simulink model "genpath_firmware"  (R2021a)
settings: Solver=FixedStepDiscrete  StartTime=0.0  StopTime=Inf  FixedStep=50e-6  RelTol=1e-3  EnableMultiTasking=on
undefined symbols (not defined in the file or in its folder): Down, GPTRIP1SEL, HW_BLDC_LQ, HW_BLDC_RS, TZ1, Up
libraries: c2802xlib x10, mcbcontrolslib x4, simulink x2, c280xlib x2, c28004xlib x2, dspstat3 x2, c2000lib x1
settings Model: SimulationMode=external  ExtModeTrigDuration=8  Creator=61301765  LastModifiedBy=61301765
settings OptimizationCC: DefaultUnderspecifiedDataType=single  EnhancedBackFolding=on  PassReuseOutputArgsAs=Individual arguments  ZeroExternalMemoryAtStartup=off  ZeroInternalMemoryAtStartup=off  MaxStackSize=1024  OptimizeBlockOrder=speed  DifferentSizesBufferReuse=on  OptimizationCustomize=off  DenormalBehavior=FlushToZero  EfficientTunableParamExpr=on
settings DebuggingCC: SignalRangeChecking=warning  ParameterPrecisionLossMsg=none  ParameterTunabilityLossMsg=error
settings HardwareCC: ProdBitPerChar=16  ProdBitPerInt=16  ProdBitPerPointer=32  ProdBitPerSizeT=32  ProdBitPerPtrDiffT=32  ProdLargestAtomicInteger=Integer  ProdLargestAtomicFloat=None  ProdWordSize=16  ProdLongLongMode=on  ProdHWDeviceType=Texas Instruments->C2000
settings SFSimCC: MATLABDynamicMemAlloc=off
settings RTWCC: SystemTargetFile=ert.tlc  HardwareBoard=TI Piccolo F280049C LaunchPad  TemplateMakefile=ert_default_tmf  Toolchain=Texas Instruments Code Composer Studio (C2000)
settings CodeAppCC: ForceParamTrailComments=on  IgnoreCustomStorageClasses=off  OperatorAnnotations=on  SimulinkDataObjDesc=on  SFDataObjDesc=on  InsertBlockDesc=on
settings ERTTargetCC: TargetLangStandard=C99 (ISO)  CodeReplacementLibrary=TI C28x  ExtModeTransport=3  ExtModeStaticAllocSize=5000

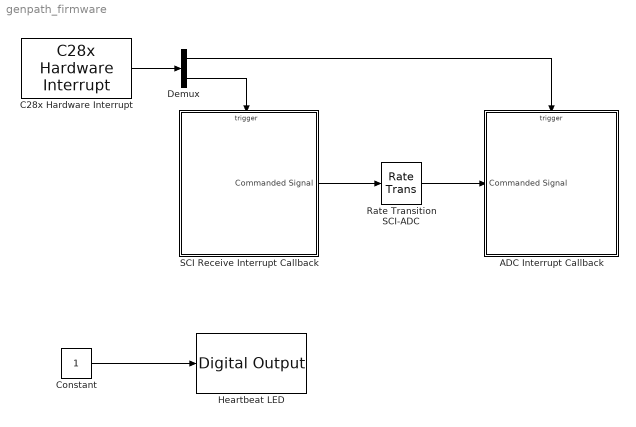
== system genpath_firmware ==
  ADC Interrupt Callback : Subsystem
  C28x Hardware Interrupt : c2000lib/Scheduling/C28x Hardware Interrupt  irqnumbers=[1 9]  pienumbers=[1 1]  irqpriorities=[30 50]  irqpreempts=[0 0]  showinput=off  dspchiptype=C280X
      settings: SourceProductBaseCode=TIC2000
  Constant : Constant  SampleTime=1
  Demux : Demux  Outputs=2
  Heartbeat LED : c28004xlib/Digital Output  GPIO_Number=GPIO16~GPIO23  GPIO_Bit0=off  GPIO_BIT0_Toggle=off  GPIO_Bit1=off  GPIO_BIT1_Toggle=off  GPIO_Bit2=off  GPIO_BIT2_Toggle=off  GPIO_Bit3=off  GPIO_BIT3_Toggle=off  GPIO_Bit4=off  GPIO_BIT4_Toggle=off  GPIO_Bit5=off  GPIO_BIT5_Toggle=off  GPIO_Bit6=off  GPIO_BIT6_Toggle=off  GPIO_Bit7=on  GPIO_BIT7_Toggle=on
      settings: SourceProductBaseCode=TIC2000
  Rate Transition SCI-ADC : RateTransition  Deterministic=off
  SCI Receive Interrupt Callback : Subsystem  TreatAsAtomicUnit=on
  wires:
  C28x Hardware Interrupt/1 -> Demux/1
  Demux/1 -> ADC Interrupt Callback/Trigger
  Demux/2 -> SCI Receive Interrupt Callback/Trigger
  SCI Receive Interrupt Callback/1(Commanded Signal) -> Rate Transition SCI-ADC/1
  Rate Transition SCI-ADC/1 -> ADC Interrupt Callback/1(Commanded Signal)
  Constant/1 -> Heartbeat LED/1

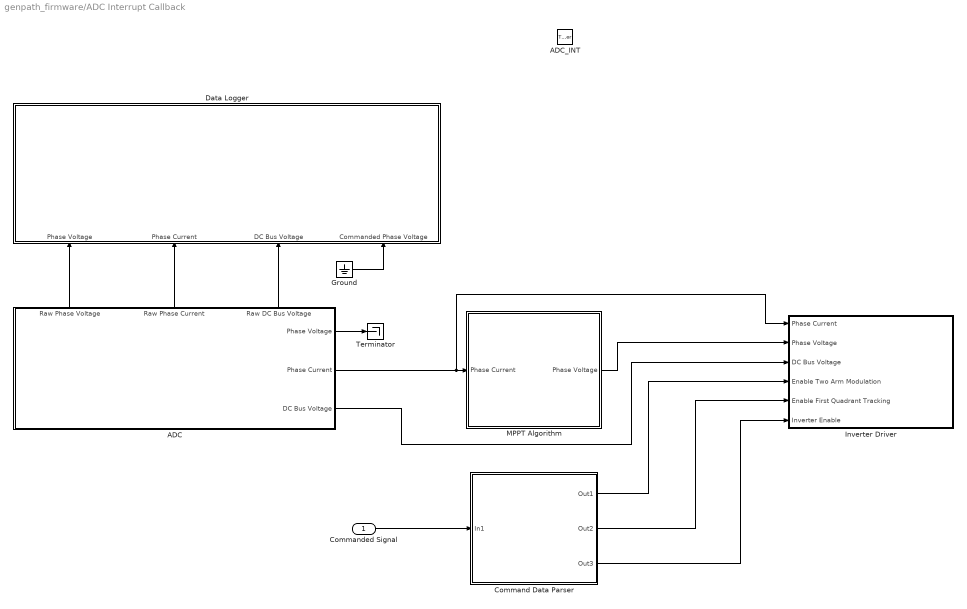
== system genpath_firmware/ADC Interrupt Callback ==
  Commanded Signal : Inport
  ADC_INT : TriggerPort  TriggerType=function-call  VariantControl=(inherit)  PortDimensions=1
  ADC : Subsystem
      settings: PortSchema="{\"entries\":[{\"content\":{\"sides\":[{\"content\":{\"connectorIds\":[]},\"type\":\"ConnectorPlacement.EquallySpacedRectSide\",\"uuid\":\"121481ca-fda4-4661-8e59-e98dfd115aae\"},{\"content\":{\"connectorIds\":[\"Out1\",\"Out2\",\"Out3\"],\"side\":\"RIGHT\"},\"type\":\"ConnectorPlacement.EquallySpacedRectSide\",\"uuid\":\"d9425efb-81e2-49c1-88ad-8da309b1ba27\"},{\"content\":{\"connectorIds\":[\"Out4\",\"Out5\",\"Out6\"],\"side\":\"TOP\"},\"type\":\"ConnectorPlacement.EquallySpacedRectSide\",\"uuid\":\"27531ece-2072-4814-ac7a-51eb1a4c9f3b\"}]},\"type\":\"ConnectorPlacement.EquallySpacedConnector\",\"uuid\":\"737147cc-a23f-43e1-a409-f74c121ac69e\"}],\"packageUris\":[\"http://schema.mathworks.com/mf0/Connector/R2020b\"],\"version\":\"1.0\"}"
  Command Data Parser : Subsystem
  Data Logger : Subsystem
      settings: PortSchema="{\"entries\":[{\"content\":{\"sides\":[{\"content\":{\"connectorIds\":[]},\"type\":\"ConnectorPlacement.EquallySpacedRectSide\",\"uuid\":\"541feeb7-3051-4b56-bc24-d8aa1f675040\"},{\"content\":{\"connectorIds\":[],\"side\":\"RIGHT\"},\"type\":\"ConnectorPlacement.EquallySpacedRectSide\",\"uuid\":\"d4df6ee5-703f-44a2-87e9-183543f9d1ff\"},{\"content\":{\"connectorIds\":[],\"side\":\"TOP\"},\"type\":\"ConnectorPlacement.EquallySpacedRectSide\",\"uuid\":\"c3c60c1a-c014-455a-bf82-8a05ef0e8309\"},{\"content\":{\"connectorIds\":[\"In1\",\"In2\",\"In3\",\"In4\"],\"side\":\"BOTTOM\"},\"type\":\"ConnectorPlacement.EquallySpacedRectSide\",\"uuid\":\"c9c2171d-b233-4586-8a06-dfee71a71187\"}]},\"type\":\"ConnectorPlacement.EquallySpacedConnector\",\"uuid\":\"cbd8768e-8563-430e-ae2e-68c4ac21817b\"}],\"packageUris\":[\"http://schema.mathworks.com/mf0/Connector/R2020b\"],\"version\":\"1.0\"}"
  Ground : Ground
  Inverter Driver : Subsystem
  MPPT Algorithm : Subsystem
  Terminator : Terminator
  wires:
  ADC/3(DC Bus Voltage) -> Inverter Driver/3(DC Bus Voltage)
  ADC/2(Phase Current) -> Inverter Driver/1(Phase Current), MPPT Algorithm/1(Phase Current)
  MPPT Algorithm/1(Phase Voltage) -> Inverter Driver/2(Phase Voltage)
  ADC/4(Raw Phase Voltage) -> Data Logger/1(Phase Voltage)
  ADC/5(Raw Phase Current) -> Data Logger/2(Phase Current)
  ADC/6(Raw DC Bus Voltage) -> Data Logger/3(DC Bus Voltage)
  Commanded Signal/1 -> Command Data Parser/1(In1)
  Command Data Parser/1(Out1) -> Inverter Driver/4(Enable Two Arm Modulation)
  Command Data Parser/2(Out2) -> Inverter Driver/5(Enable First Quadrant Tracking)
  Command Data Parser/3(Out3) -> Inverter Driver/6(Inverter Enable)
  Ground/1 -> Data Logger/4(Commanded Phase Voltage)
  ADC/1(Phase Voltage) -> Terminator/1

== system genpath_firmware/SCI Receive Interrupt Callback ==
  SCI_RX_INT : TriggerPort  TriggerType=function-call  VariantControl=(inherit)
  SCIA Receive : c280xlib/SCI Receive  sciModule=A  dataHead='S'  dataTail='E'  dataType=single  dataDim=3  initValue=0  errOption=Output the last received value  errValue=0  sampleTime=-1  outputStatus=off  postInterrupt=on  numFifo=6
      settings: SourceProductBaseCode=TIC2000
  Commanded Signal : Outport
  wires:
  SCIA Receive/1 -> Commanded Signal/1

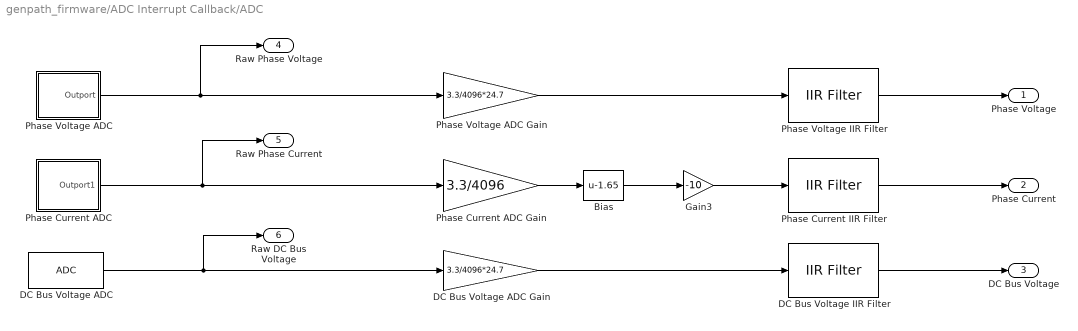
== system genpath_firmware/ADC Interrupt Callback/ADC ==
  Bias : Bias  Bias=-1.65
  DC Bus Voltage ADC : c2802xlib/ADC  blkParamProc=C2000_Type5  ADCModule=A  samplingMode=Single sample mode  ADCResolution=12-bit (Single-ended input)  useSOC1=SOC6  useSOC2=SOC0_SOC1  SOCAcquisitionWindow=8  SOCTriggerSource=ePWM1_ADCSOCA  SOCInterruptTrigger=No ADCINT  Ts=-1  dType=uint16  postInterrupt=on  interruptSel=ADCINT1  ADCINTContinuous=on  endma=off  chdma=1  conv1=ADCINA0  conv2=ADCINA0 and ADCINB0  conv1_Type4=ADCIN6  conv2_Type4=ADCIN0 and ADCIN1
  DC Bus Voltage ADC Gain : Gain  Gain=3.3/4096*24.7  OutDataTypeStr=single
  DC Bus Voltage IIR Filter : mcbcontrolslib/IIR Filter  VariantControl=Low Pass Filter  VariantSelect=Low-pass  Filter_constant=0.02  advancedSettings=on  Ts=50e-6  cutOff_freq=64.9612
      settings: SourceProductBaseCode=MT
  Gain3 : Gain  Gain=-10
  Phase Current ADC : Subsystem
  Phase Current ADC Gain : Gain  Gain=3.3/4096  OutDataTypeStr=single
  Phase Current IIR Filter : mcbcontrolslib/IIR Filter  VariantControl=Low Pass Filter  VariantSelect=Low-pass  Filter_constant=0.02  advancedSettings=on  Ts=50e-6  cutOff_freq=64.9612
      settings: SourceProductBaseCode=MT
  Phase Voltage ADC : Subsystem
  Phase Voltage ADC Gain : Gain  Gain=3.3/4096*24.7  OutDataTypeStr=single
  Phase Voltage IIR Filter : mcbcontrolslib/IIR Filter  VariantControl=Low Pass Filter  VariantSelect=Low-pass  Filter_constant=0.5  advancedSettings=on  Ts=50e-6  cutOff_freq=3183.0989
      settings: SourceProductBaseCode=MT
  Phase Voltage : Outport  Unit=V
  Phase Current : Outport  Port=2  Unit=A
  DC Bus Voltage : Outport  Port=3  Unit=V
  Raw Phase Voltage : Outport  Port=4
  Raw Phase Current : Outport  Port=5
  Raw DC Bus Voltage : Outport  Port=6
  wires:
  Phase Current ADC Gain/1 -> Bias/1
  Phase Current ADC/1(Outport1) -> Raw Phase Current/1, Phase Current ADC Gain/1
  Gain3/1 -> Phase Current IIR Filter/1
  DC Bus Voltage ADC/1 -> Raw DC Bus Voltage/1, DC Bus Voltage ADC Gain/1
  Phase Voltage ADC/1(Outport) -> Raw Phase Voltage/1, Phase Voltage ADC Gain/1
  Bias/1 -> Gain3/1
  Phase Voltage ADC Gain/1 -> Phase Voltage IIR Filter/1
  DC Bus Voltage IIR Filter/1 -> DC Bus Voltage/1
  DC Bus Voltage ADC Gain/1 -> DC Bus Voltage IIR Filter/1
  Phase Current IIR Filter/1 -> Phase Current/1
  Phase Voltage IIR Filter/1 -> Phase Voltage/1

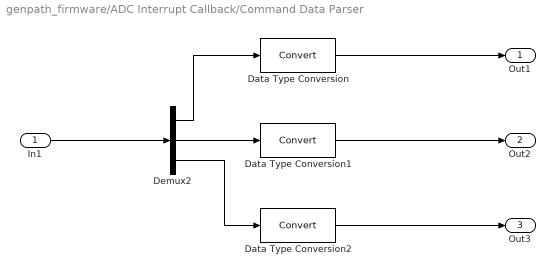
== system genpath_firmware/ADC Interrupt Callback/Command Data Parser ==
  In1 : Inport
  Data Type Conversion : DataTypeConversion
  Data Type Conversion1 : DataTypeConversion
  Data Type Conversion2 : DataTypeConversion
  Demux2 : Demux  Outputs=3
  Out1 : Outport
  Out2 : Outport  Port=2
  Out3 : Outport  Port=3
  wires:
  Demux2/1 -> Data Type Conversion/1
  Demux2/2 -> Data Type Conversion1/1
  In1/1 -> Demux2/1
  Demux2/3 -> Data Type Conversion2/1
  Data Type Conversion/1 -> Out1/1
  Data Type Conversion1/1 -> Out2/1
  Data Type Conversion2/1 -> Out3/1

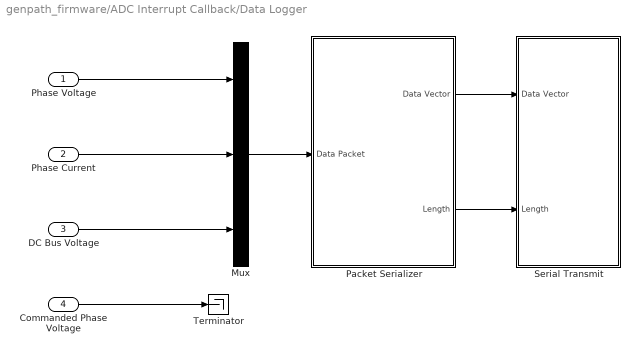
== system genpath_firmware/ADC Interrupt Callback/Data Logger ==
  Phase Voltage : Inport
  Phase Current : Inport  Port=2
  DC Bus Voltage : Inport  Port=3
  Commanded Phase Voltage : Inport  Port=4
  Mux : Mux  Inputs=3
  Packet Serializer : Subsystem
  Serial Transmit : Subsystem  TreatAsAtomicUnit=on
  Terminator : Terminator
  wires:
  Mux/1 -> Packet Serializer/1(Data Packet)
  Packet Serializer/2(Length) -> Serial Transmit/2(Length)
  Packet Serializer/1(Data Vector) -> Serial Transmit/1(Data Vector)
  Phase Voltage/1 -> Mux/1
  Phase Current/1 -> Mux/2
  DC Bus Voltage/1 -> Mux/3
  Commanded Phase Voltage/1 -> Terminator/1

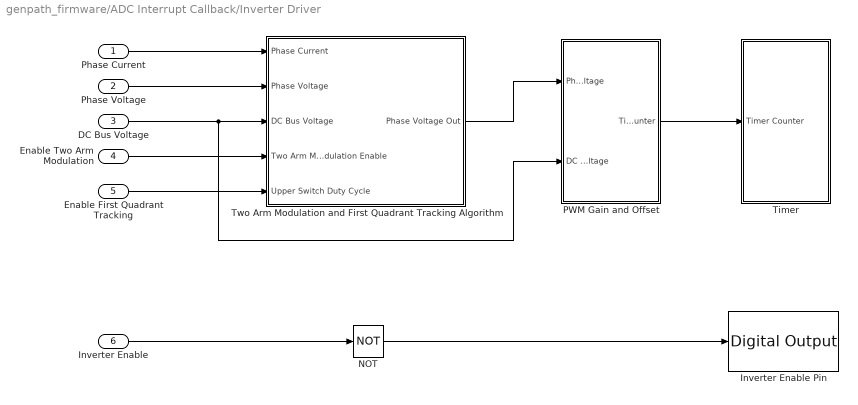
== system genpath_firmware/ADC Interrupt Callback/Inverter Driver ==
  Phase Current : Inport
  Phase Voltage : Inport  Port=2
  DC Bus Voltage : Inport  Port=3
  Enable Two Arm Modulation : Inport  Port=4  OutDataTypeStr=boolean
  Enable First Quadrant Tracking : Inport  Port=5
  Inverter Enable : Inport  Port=6
  Inverter Enable Pin : c28004xlib/Digital Output  GPIO_Number=GPIO32~GPIO39  GPIO_Bit0=off  GPIO_BIT0_Toggle=off  GPIO_Bit1=on  GPIO_BIT1_Toggle=off  GPIO_Bit2=off  GPIO_BIT2_Toggle=off  GPIO_Bit3=off  GPIO_BIT3_Toggle=off  GPIO_Bit4=off  GPIO_BIT4_Toggle=off  GPIO_Bit5=off  GPIO_BIT5_Toggle=off  GPIO_Bit6=off  GPIO_BIT6_Toggle=off  GPIO_Bit7=off  GPIO_BIT7_Toggle=off
      settings: SourceProductBaseCode=TIC2000
  NOT : Logic  Operator=NOT  IconShape=distinctive  AllPortsSameDT=off  OutDataTypeStr=boolean
  PWM Gain and Offset : Subsystem
  Timer : Subsystem
  Two Arm Modulation and First Quadrant Tracking Algorithm : Subsystem
  wires:
  DC Bus Voltage/1 -> Two Arm Modulation and First Quadrant Tracking Algorithm/3(DC Bus Voltage), PWM Gain and Offset/2(DC Bus Voltage)
  Phase Voltage/1 -> Two Arm Modulation and First Quadrant Tracking Algorithm/2(Phase Voltage)
  Enable Two Arm Modulation/1 -> Two Arm Modulation and First Quadrant Tracking Algorithm/4(Two Arm Modulation Enable)
  Enable First Quadrant Tracking/1 -> Two Arm Modulation and First Quadrant Tracking Algorithm/5(Upper Switch Duty Cycle)
  Two Arm Modulation and First Quadrant Tracking Algorithm/1(Phase Voltage Out) -> PWM Gain and Offset/1(Phase Voltage)
  NOT/1 -> Inverter Enable Pin/1
  Inverter Enable/1 -> NOT/1
  PWM Gain and Offset/1(Timer Counter) -> Timer/1(Timer Counter)
  Phase Current/1 -> Two Arm Modulation and First Quadrant Tracking Algorithm/1(Phase Current)

== system genpath_firmware/ADC Interrupt Callback/MPPT Algorithm ==
  Phase Current : Inport
  Derivative : Subsystem  Commented=on
  Gain1 : Gain  Gain=-HW_BLDC_RS
  Gain2 : Gain  Commented=on  Gain=-HW_BLDC_LQ
  IIR Filter : mcbcontrolslib/IIR Filter  Commented=on  VariantControl=Low Pass Filter  VariantSelect=Low-pass  Filter_constant=0.1  advancedSettings=on  Ts=100e-6  cutOff_freq=176.8388
      settings: SourceProductBaseCode=MT
  Sum : Sum  Inputs=|++
  Phase Voltage : Outport
  wires:
  Phase Current/1 -> Gain2/1, Gain1/1
  Gain1/1 -> Phase Voltage/1, Sum/1
  IIR Filter/1 -> Sum/2
  Gain2/1 -> Derivative/1(In3)
  Derivative/1(Out1) -> IIR Filter/1

== system genpath_firmware/ADC Interrupt Callback/ADC/Phase Current ADC ==
  Bias : Bias  Bias=+5  SaturateOnIntegerOverflow=on
  Bias1 : Bias  Bias=+5  SaturateOnIntegerOverflow=on
  Bias2 : Bias  Bias=+5  SaturateOnIntegerOverflow=on
  I_A : c2802xlib/ADC  blkParamProc=C2000_Type5  ADCModule=C  samplingMode=Single sample mode  ADCResolution=12-bit (Single-ended input)  useSOC1=SOC3  useSOC2=SOC0_SOC1  SOCAcquisitionWindow=8  SOCTriggerSource=ePWM1_ADCSOCA  SOCInterruptTrigger=No ADCINT  Ts=-1  dType=uint16  postInterrupt=off  interruptSel=ADCINT1  ADCINTContinuous=on  endma=off  chdma=1  conv1=ADCINA0  conv2=ADCINA0 and ADCINB0  conv1_Type4=ADCIN3  conv2_Type4=ADCIN0 and ADCIN1
  I_B : c2802xlib/ADC  blkParamProc=C2000_Type5  ADCModule=C  samplingMode=Single sample mode  ADCResolution=12-bit (Single-ended input)  useSOC1=SOC4  useSOC2=SOC0_SOC1  SOCAcquisitionWindow=8  SOCTriggerSource=ePWM1_ADCSOCA  SOCInterruptTrigger=No ADCINT  Ts=-1  dType=uint16  postInterrupt=off  interruptSel=ADCINT1  ADCINTContinuous=on  endma=off  chdma=1  conv1=ADCINA0  conv2=ADCINA0 and ADCINB0  conv1_Type4=ADCIN5  conv2_Type4=ADCIN0 and ADCIN1
  I_C : c2802xlib/ADC  blkParamProc=C2000_Type5  ADCModule=A  samplingMode=Single sample mode  ADCResolution=12-bit (Single-ended input)  useSOC1=SOC5  useSOC2=SOC0_SOC1  SOCAcquisitionWindow=8  SOCTriggerSource=ePWM1_ADCSOCA  SOCInterruptTrigger=No ADCINT  Ts=-1  dType=uint16  postInterrupt=off  interruptSel=ADCINT1  ADCINTContinuous=on  endma=off  chdma=1  conv1=ADCINA0  conv2=ADCINA0 and ADCINB0  conv1_Type4=ADCIN3  conv2_Type4=ADCIN0 and ADCIN1
  Mux1 : Mux  Inputs=3
  Outport1 : Outport
  wires:
  Mux1/1 -> Outport1/1
  I_A/1 -> Bias/1
  I_B/1 -> Bias1/1
  I_C/1 -> Bias2/1
  Bias1/1 -> Mux1/2
  Bias/1 -> Mux1/1
  Bias2/1 -> Mux1/3

== system genpath_firmware/ADC Interrupt Callback/ADC/Phase Voltage ADC ==
  Mux1 : Mux  Inputs=3
  V_A : c2802xlib/ADC  blkParamProc=C2000_Type5  ADCModule=B  samplingMode=Single sample mode  ADCResolution=12-bit (Single-ended input)  useSOC1=SOC0  useSOC2=SOC0_SOC1  SOCAcquisitionWindow=8  SOCTriggerSource=ePWM1_ADCSOCA  SOCInterruptTrigger=No ADCINT  Ts=-1  dType=uint16  postInterrupt=off  interruptSel=ADCINT1  ADCINTContinuous=on  endma=off  chdma=1  conv1=ADCINA0  conv2=ADCINA0 and ADCINB0  conv1_Type4=ADCIN6  conv2_Type4=ADCIN0 and ADCIN1
  V_B : c2802xlib/ADC  blkParamProc=C2000_Type5  ADCModule=C  samplingMode=Single sample mode  ADCResolution=12-bit (Single-ended input)  useSOC1=SOC1  useSOC2=SOC0_SOC1  SOCAcquisitionWindow=8  SOCTriggerSource=ePWM1_ADCSOCA  SOCInterruptTrigger=No ADCINT  Ts=-1  dType=uint16  postInterrupt=off  interruptSel=ADCINT1  ADCINTContinuous=on  endma=off  chdma=1  conv1=ADCINA0  conv2=ADCINA0 and ADCINB0  conv1_Type4=ADCIN14  conv2_Type4=ADCIN0 and ADCIN1
  V_C : c2802xlib/ADC  blkParamProc=C2000_Type5  ADCModule=C  samplingMode=Single sample mode  ADCResolution=12-bit (Single-ended input)  useSOC1=SOC2  useSOC2=SOC0_SOC1  SOCAcquisitionWindow=8  SOCTriggerSource=ePWM1_ADCSOCA  SOCInterruptTrigger=No ADCINT  Ts=-1  dType=uint16  postInterrupt=off  interruptSel=ADCINT1  ADCINTContinuous=on  endma=off  chdma=1  conv1=ADCINA0  conv2=ADCINA0 and ADCINB0  conv1_Type4=ADCIN1  conv2_Type4=ADCIN0 and ADCIN1
  Outport : Outport
  wires:
  Mux1/1 -> Outport/1
  V_B/1 -> Mux1/2
  V_A/1 -> Mux1/1
  V_C/1 -> Mux1/3

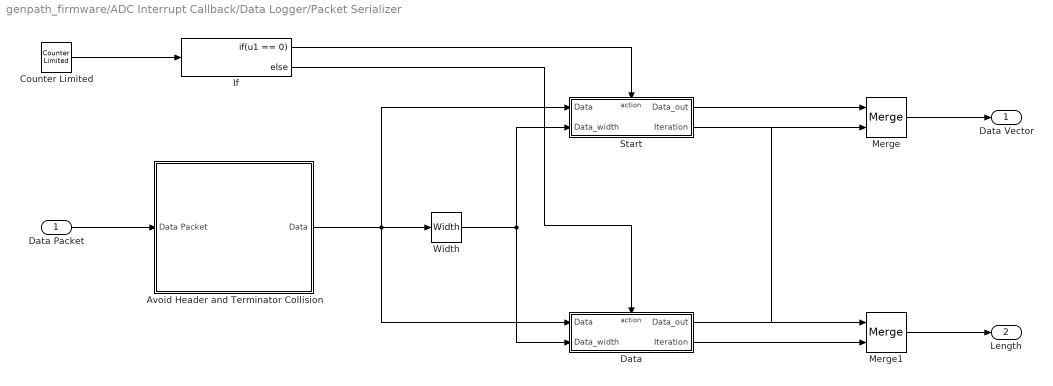
== system genpath_firmware/ADC Interrupt Callback/Data Logger/Packet Serializer ==
  Data Packet : Inport
  Avoid Header and Terminator Collision : Subsystem  TreatAsAtomicUnit=on
  Counter Limited : simulink/Sources/Counter Limited  uplimit=999  tsamp=-1
  Data : Subsystem  TreatAsAtomicUnit=on
  If : If  IfExpression=u1 == 0
  Merge : Merge
  Merge1 : Merge
  Start : Subsystem  TreatAsAtomicUnit=on
  Width : Width  DataType=uint16
  Data Vector : Outport
  Length : Outport  Port=2
  wires:
  Data/2(Iteration) -> Merge1/2
  Data Packet/1 -> Avoid Header and Terminator Collision/1(Data Packet)
  If/2 -> Data/Action
  Start/2(Iteration) -> Merge1/1
  Width/1 -> Data/2(Data_width), Start/2(Data_width)
  Counter Limited/1 -> If/1
  Merge1/1 -> Length/1
  If/1 -> Start/Action
  Data/1(Data_out) -> Merge/2
  Start/1(Data_out) -> Merge/1
  Merge/1 -> Data Vector/1
  Avoid Header and Terminator Collision/1(Data) -> Start/1(Data), Width/1, Data/1(Data)

== system genpath_firmware/ADC Interrupt Callback/Data Logger/Serial Transmit ==
  Data Vector : Inport
  Length : Inport  Port=2
  Add : Sum  Inputs=+-  OutDataTypeStr=Inherit: Same as first input
  Index Vector : MultiPortSwitch  Inputs=1
  SCIA Transmit : c280xlib/SCI Transmit  sciModule=A  dataHead=''  dataTail=''  postInterrupt=off  numFifo=1
  While Data Available : WhileIterator  MaxIters=-1  WhileBlockType=do-while  ShowIterationPort=on  OutputDataType=int16
  wires:
  Length/1 -> Add/1
  Add/1 -> While Data Available/1
  Data Vector/1 -> Index Vector/2
  While Data Available/1 -> Index Vector/1, Add/2
  Index Vector/1 -> SCIA Transmit/1

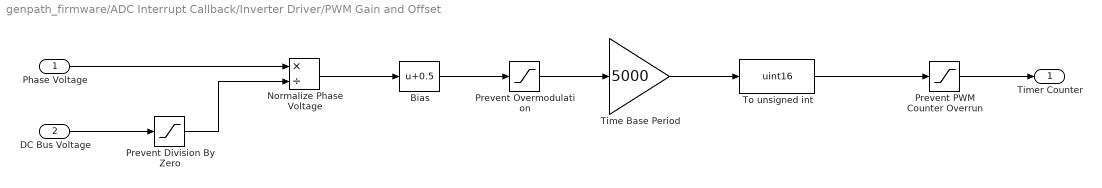
== system genpath_firmware/ADC Interrupt Callback/Inverter Driver/PWM Gain and Offset ==
  Phase Voltage : Inport
  DC Bus Voltage : Inport  Port=2
  Bias : Bias  Bias=0.5
  Normalize Phase Voltage : Product  Inputs=*/
  Prevent Division By Zero : Saturate  UpperLimit=81.5  LowerLimit=0.1
  Prevent Overmodulation : Saturate  UpperLimit=1  LowerLimit=0
  Prevent PWM Counter Overrun : Saturate  UpperLimit=4995  LowerLimit=0
  Time Base Period : Gain  Gain=5000
  To unsigned int : DataTypeConversion  OutDataTypeStr=uint16  ConvertRealWorld=Stored Integer (SI)  SaturateOnIntegerOverflow=on
  Timer Counter : Outport
  wires:
  Normalize Phase Voltage/1 -> Bias/1
  Prevent Division By Zero/1 -> Normalize Phase Voltage/2
  Phase Voltage/1 -> Normalize Phase Voltage/1
  DC Bus Voltage/1 -> Prevent Division By Zero/1
  Bias/1 -> Prevent Overmodulation/1
  Prevent Overmodulation/1 -> Time Base Period/1
  Time Base Period/1 -> To unsigned int/1
  Prevent PWM Counter Overrun/1 -> Timer Counter/1
  To unsigned int/1 -> Prevent PWM Counter Overrun/1

== system genpath_firmware/ADC Interrupt Callback/Inverter Driver/Timer ==
  Timer Counter : Inport
  Demux : Demux  Outputs=3
  SW_A : c2802xlib/ePWM  PwmType=C2000_Type4  useModule=ePWM1  ePWMxLINKTBPRD=Not Linked  periodUnits=Clock cycles  timerSource=Specify via dialog  timerPeriod_clk=5000  timerPeriod_sec=0.0001  tbshadow=Counter equals to zero  countingMode=Up-Down  phaseActiveEnable=Disable  phaseDirection=Count down after sync  phaseActive=0  synchronizationEnable=off  dcaevt1Sync=off  dcbevt1Sync=off  synchronizationOption=Disable  perSynchronizationOption=Counter equals to period (CTR=PRD)  clockPrescale=1  HSclockPrescale=1  enswap=off  ePWMxAStatus=on  ePWMxAactionLogic1=Set  ePWMxAactionLogic2=Clear  ePWMxAactionLogic3=Clear  ePWMxAactionLogic4=Set  ePWMxAactionLogic5=Do nothing  ePWMxAactionLogic6=Do nothing  ePWMxACSFenable=off  ePWMxACSFvalue=Forcing disable  ePWMxASFreload=Zero  ePWMxBStatus=off  ePWMxBactionLogic1=Set  ePWMxBactionLogic2=Clear  ePWMxBactionLogic3=Do nothing  ePWMxBactionLogic4=Do nothing  ePWMxBactionLogic5=Clear  ePWMxBactionLogic6=Set  ePWMxBCSFenable=off  ePWMxBCSFvalue=Forcing disable  ePWMxBSFreload=Zero  ePWNxBOutWay=off  ePWMxLINKCMPA=Not Linked  CMPAUnits=Clock cycles  CMPASource=Input port  CMPAValue_per=50  CMPAValue_clk=0  enCMPAshadow=Counter equals to zero (CTR=Zero)  ePWMxLINKCMPB=Not Linked  CMPBUnits=Clock cycles  CMPBSource=Specify via dialog  CMPBValue_per=50  CMPBValue_clk=32000  enCMPBshadow=Counter equals to zero (CTR=Zero)  ePWMxLINKCMPC=Not Linked  CMPCUnits=Clock cycles  CMPCSource=Specify via dialog  CMPCValue_per=50  CMPCValue_clk=32000  enCMPCshadow=Counter equals to zero (CTR=Zero)  ePWMxLINKCMPD=Not Linked  CMPDUnits=Clock cycles  CMPDSource=Specify via dialog  CMPDValue_per=50  CMPDValue_clk=32000  enCMPDshadow=Counter equals to zero (CTR=Zero)  enableDBePWMxA=on  enableDBePWMxB=on  enhalfcycle=off  DBpolarity=Active high complementary (AHC)  DBedgeDelay=Positive  DBSource_ePWMxA=ePWMxA  DBSource_ePWMxB=ePWMxA  DBPeriodUnits=Clock cycles  DBperiodSource=Specify via dialog  REDperiod=5  FEDperiod=5  REDperiod_sec=0  FEDperiod_sec=0  LoadModeDBRED=Immediate without using shadow  LoadModeDBFED=Immediate without using shadow  adcstartModuleA=on  adcrequestEventA=First event  adcstartEventA=Digital Compare Module A Event 1 start of conversion (DCAEVT1.soc)  adcstartEventA_type2=Counter equals to period (CTR=PRD)  adcstartModuleB=off  adcrequestEventB=First event  adcstartEventB=Counter equals to zero (CTR=Zero)  adcstartEventB_type2=Counter equals to zero (CTR=Zero)  intEn=off  intPrd=First event  intSel=Counter equals to zero (CTR=Zero)  intSel_type2=Counter equals to zero (CTR=Zero)  hrpe=off  enHRPWM=off  HRPWM_LoadMode=Counter equals to period (CTR=PRD)  HRPWM_CTLMode=Duty or Period control mode  HRPWM_EDGMode=Both edge  hrpeb=off  enHRPWMB=off  HRPWM_LoadModeB=Counter equals to zero (CTR=ZERO)  HRPWM_CTLModeB=Duty or Period control mode  HRPWM_EDGModeB=Both edge  enHRDBRED=off  enHRDBFED=off  enSFO=on  enautoconv=on  chopperEnable=off  chopperFrequency=1  chopperFirstwidth=1  chopperDuty=12.5%  tripZonesource=Specify via dialog  tzselOSHT1=off  tzselOSHT2=off  tzselOSHT3=off  tzselOSHDCAEV1=off  tzselOSHDCBEV1=off  tzselCBC1=off  tzselCBC2=off  tzselCBC3=off  tzselCBCDCAEV2=off  tzselCBCDCBEV2=off  tzselOSHT4=off  tzselOSHT5=off  tzselOSHT6=off  tzselCBC4=off  tzselCBC5=off  tzselCBC6=off  enTzOstIntr=off  enTzCbcIntr=off  enTzDCAEVT1Intr=off  enTzDCAEVT2Intr=off  enTzDCBEVT1Intr=off  enTzDCBEVT2Intr=off  ePWMxAforced=No action  ePWMxBforced=No action  DCAEVT1forced=No action  DCBEVT1forced=No action  DCAEVT2forced=No action  DCBEVT2forced=No action  dcah=Trip Zone 1 input (TZ1)  dcal=Trip Zone 2 input (TZ2)  dcbh=Trip Zone 1 input (TZ1)  dcbl=Trip Zone 2 input (TZ2)  dcah_type2=GPTRIP1SEL/(TZ1)  dcal_type2=GPTRIP1SEL/(TZ1)  dcbh_type2=GPTRIP1SEL/(TZ1)  dcbl_type2=GPTRIP1SEL/(TZ1)  gendcaevt1=Event disabled  gendcaevt2=Event disabled  gendcbevt1=Event disabled  gendcbevt2=Event disabled  dcaevt1src=DCAEVT1 with sync  dcaevt2src=DCAEVT2 with sync  dcbevt1src=DCBEVT1 with sync  dcbevt2src=DCBEVT2 with sync  pulsesel=Counter equals to zero (CTR=Zero)  blankinv=off  blankoffset=0  blankwidth=0  evsrcsel=Filtered version of DCAEVT1 (DCAEVT1FILT)  encape=off
  SW_B : c2802xlib/ePWM  PwmType=C2000_Type4  useModule=ePWM4  ePWMxLINKTBPRD=ePWM1  periodUnits=Clock cycles  timerSource=Specify via dialog  timerPeriod_clk=5000  timerPeriod_sec=0.0001  tbshadow=Counter equals to zero  countingMode=Up-Down  phaseActiveEnable=Disable  phaseDirection=Count down after sync  phaseActive=0  synchronizationEnable=off  dcaevt1Sync=off  dcbevt1Sync=off  synchronizationOption=Disable  perSynchronizationOption=Counter equals to period (CTR=PRD)  clockPrescale=1  HSclockPrescale=1  enswap=off  ePWMxAStatus=on  ePWMxAactionLogic1=Set  ePWMxAactionLogic2=Clear  ePWMxAactionLogic3=Clear  ePWMxAactionLogic4=Set  ePWMxAactionLogic5=Do nothing  ePWMxAactionLogic6=Do nothing  ePWMxACSFenable=off  ePWMxACSFvalue=Forcing disable  ePWMxASFreload=Zero  ePWMxBStatus=off  ePWMxBactionLogic1=Set  ePWMxBactionLogic2=Clear  ePWMxBactionLogic3=Do nothing  ePWMxBactionLogic4=Do nothing  ePWMxBactionLogic5=Clear  ePWMxBactionLogic6=Set  ePWMxBCSFenable=off  ePWMxBCSFvalue=Forcing disable  ePWMxBSFreload=Zero  ePWNxBOutWay=off  ePWMxLINKCMPA=Not Linked  CMPAUnits=Clock cycles  CMPASource=Input port  CMPAValue_per=50  CMPAValue_clk=0  enCMPAshadow=Counter equals to zero (CTR=Zero)  ePWMxLINKCMPB=Not Linked  CMPBUnits=Clock cycles  CMPBSource=Specify via dialog  CMPBValue_per=50  CMPBValue_clk=32000  enCMPBshadow=Counter equals to zero (CTR=Zero)  ePWMxLINKCMPC=Not Linked  CMPCUnits=Clock cycles  CMPCSource=Specify via dialog  CMPCValue_per=50  CMPCValue_clk=32000  enCMPCshadow=Counter equals to zero (CTR=Zero)  ePWMxLINKCMPD=Not Linked  CMPDUnits=Clock cycles  CMPDSource=Specify via dialog  CMPDValue_per=50  CMPDValue_clk=32000  enCMPDshadow=Counter equals to zero (CTR=Zero)  enableDBePWMxA=on  enableDBePWMxB=on  enhalfcycle=off  DBpolarity=Active high complementary (AHC)  DBedgeDelay=Positive  DBSource_ePWMxA=ePWMxA  DBSource_ePWMxB=ePWMxA  DBPeriodUnits=Clock cycles  DBperiodSource=Specify via dialog  REDperiod=5  FEDperiod=5  REDperiod_sec=0  FEDperiod_sec=0  LoadModeDBRED=Immediate without using shadow  LoadModeDBFED=Immediate without using shadow  adcstartModuleA=on  adcrequestEventA=First event  adcstartEventA=Digital Compare Module A Event 1 start of conversion (DCAEVT1.soc)  adcstartEventA_type2=Counter equals to period (CTR=PRD)  adcstartModuleB=off  adcrequestEventB=First event  adcstartEventB=Counter equals to zero (CTR=Zero)  adcstartEventB_type2=Counter equals to zero (CTR=Zero)  intEn=off  intPrd=First event  intSel=Counter equals to zero (CTR=Zero)  intSel_type2=Counter equals to zero (CTR=Zero)  hrpe=off  enHRPWM=off  HRPWM_LoadMode=Counter equals to period (CTR=PRD)  HRPWM_CTLMode=Duty or Period control mode  HRPWM_EDGMode=Both edge  hrpeb=off  enHRPWMB=off  HRPWM_LoadModeB=Counter equals to zero (CTR=ZERO)  HRPWM_CTLModeB=Duty or Period control mode  HRPWM_EDGModeB=Both edge  enHRDBRED=off  enHRDBFED=off  enSFO=on  enautoconv=on  chopperEnable=off  chopperFrequency=1  chopperFirstwidth=1  chopperDuty=12.5%  tripZonesource=Specify via dialog  tzselOSHT1=off  tzselOSHT2=off  tzselOSHT3=off  tzselOSHDCAEV1=off  tzselOSHDCBEV1=off  tzselCBC1=off  tzselCBC2=off  tzselCBC3=off  tzselCBCDCAEV2=off  tzselCBCDCBEV2=off  tzselOSHT4=off  tzselOSHT5=off  tzselOSHT6=off  tzselCBC4=off  tzselCBC5=off  tzselCBC6=off  enTzOstIntr=off  enTzCbcIntr=off  enTzDCAEVT1Intr=off  enTzDCAEVT2Intr=off  enTzDCBEVT1Intr=off  enTzDCBEVT2Intr=off  ePWMxAforced=No action  ePWMxBforced=No action  DCAEVT1forced=No action  DCBEVT1forced=No action  DCAEVT2forced=No action  DCBEVT2forced=No action  dcah=Trip Zone 1 input (TZ1)  dcal=Trip Zone 2 input (TZ2)  dcbh=Trip Zone 1 input (TZ1)  dcbl=Trip Zone 2 input (TZ2)  dcah_type2=GPTRIP1SEL/(TZ1)  dcal_type2=GPTRIP1SEL/(TZ1)  dcbh_type2=GPTRIP1SEL/(TZ1)  dcbl_type2=GPTRIP1SEL/(TZ1)  gendcaevt1=Event disabled  gendcaevt2=Event disabled  gendcbevt1=Event disabled  gendcbevt2=Event disabled  dcaevt1src=DCAEVT1 with sync  dcaevt2src=DCAEVT2 with sync  dcbevt1src=DCBEVT1 with sync  dcbevt2src=DCBEVT2 with sync  pulsesel=Counter equals to zero (CTR=Zero)  blankinv=off  blankoffset=0  blankwidth=0  evsrcsel=Filtered version of DCAEVT1 (DCAEVT1FILT)  encape=off
  SW_C : c2802xlib/ePWM  PwmType=C2000_Type4  useModule=ePWM2  ePWMxLINKTBPRD=ePWM1  periodUnits=Clock cycles  timerSource=Specify via dialog  timerPeriod_clk=5000  timerPeriod_sec=0.0001  tbshadow=Counter equals to zero  countingMode=Up-Down  phaseActiveEnable=Disable  phaseDirection=Count down after sync  phaseActive=0  synchronizationEnable=off  dcaevt1Sync=off  dcbevt1Sync=off  synchronizationOption=Disable  perSynchronizationOption=Counter equals to period (CTR=PRD)  clockPrescale=1  HSclockPrescale=1  enswap=off  ePWMxAStatus=on  ePWMxAactionLogic1=Set  ePWMxAactionLogic2=Clear  ePWMxAactionLogic3=Clear  ePWMxAactionLogic4=Set  ePWMxAactionLogic5=Do nothing  ePWMxAactionLogic6=Do nothing  ePWMxACSFenable=off  ePWMxACSFvalue=Forcing disable  ePWMxASFreload=Zero  ePWMxBStatus=off  ePWMxBactionLogic1=Set  ePWMxBactionLogic2=Clear  ePWMxBactionLogic3=Do nothing  ePWMxBactionLogic4=Do nothing  ePWMxBactionLogic5=Clear  ePWMxBactionLogic6=Set  ePWMxBCSFenable=off  ePWMxBCSFvalue=Forcing disable  ePWMxBSFreload=Zero  ePWNxBOutWay=off  ePWMxLINKCMPA=Not Linked  CMPAUnits=Clock cycles  CMPASource=Input port  CMPAValue_per=50  CMPAValue_clk=0  enCMPAshadow=Counter equals to zero (CTR=Zero)  ePWMxLINKCMPB=Not Linked  CMPBUnits=Clock cycles  CMPBSource=Specify via dialog  CMPBValue_per=50  CMPBValue_clk=32000  enCMPBshadow=Counter equals to zero (CTR=Zero)  ePWMxLINKCMPC=Not Linked  CMPCUnits=Clock cycles  CMPCSource=Specify via dialog  CMPCValue_per=50  CMPCValue_clk=32000  enCMPCshadow=Counter equals to zero (CTR=Zero)  ePWMxLINKCMPD=Not Linked  CMPDUnits=Clock cycles  CMPDSource=Specify via dialog  CMPDValue_per=50  CMPDValue_clk=32000  enCMPDshadow=Counter equals to zero (CTR=Zero)  enableDBePWMxA=on  enableDBePWMxB=on  enhalfcycle=off  DBpolarity=Active high complementary (AHC)  DBedgeDelay=Positive  DBSource_ePWMxA=ePWMxA  DBSource_ePWMxB=ePWMxA  DBPeriodUnits=Clock cycles  DBperiodSource=Specify via dialog  REDperiod=5  FEDperiod=5  REDperiod_sec=0  FEDperiod_sec=0  LoadModeDBRED=Immediate without using shadow  LoadModeDBFED=Immediate without using shadow  adcstartModuleA=on  adcrequestEventA=First event  adcstartEventA=Digital Compare Module A Event 1 start of conversion (DCAEVT1.soc)  adcstartEventA_type2=Counter equals to period (CTR=PRD)  adcstartModuleB=off  adcrequestEventB=First event  adcstartEventB=Counter equals to zero (CTR=Zero)  adcstartEventB_type2=Counter equals to zero (CTR=Zero)  intEn=off  intPrd=First event  intSel=Counter equals to zero (CTR=Zero)  intSel_type2=Counter equals to zero (CTR=Zero)  hrpe=off  enHRPWM=off  HRPWM_LoadMode=Counter equals to period (CTR=PRD)  HRPWM_CTLMode=Duty or Period control mode  HRPWM_EDGMode=Both edge  hrpeb=off  enHRPWMB=off  HRPWM_LoadModeB=Counter equals to zero (CTR=ZERO)  HRPWM_CTLModeB=Duty or Period control mode  HRPWM_EDGModeB=Both edge  enHRDBRED=off  enHRDBFED=off  enSFO=on  enautoconv=on  chopperEnable=off  chopperFrequency=1  chopperFirstwidth=1  chopperDuty=12.5%  tripZonesource=Specify via dialog  tzselOSHT1=off  tzselOSHT2=off  tzselOSHT3=off  tzselOSHDCAEV1=off  tzselOSHDCBEV1=off  tzselCBC1=off  tzselCBC2=off  tzselCBC3=off  tzselCBCDCAEV2=off  tzselCBCDCBEV2=off  tzselOSHT4=off  tzselOSHT5=off  tzselOSHT6=off  tzselCBC4=off  tzselCBC5=off  tzselCBC6=off  enTzOstIntr=off  enTzCbcIntr=off  enTzDCAEVT1Intr=off  enTzDCAEVT2Intr=off  enTzDCBEVT1Intr=off  enTzDCBEVT2Intr=off  ePWMxAforced=No action  ePWMxBforced=No action  DCAEVT1forced=No action  DCBEVT1forced=No action  DCAEVT2forced=No action  DCBEVT2forced=No action  dcah=Trip Zone 1 input (TZ1)  dcal=Trip Zone 2 input (TZ2)  dcbh=Trip Zone 1 input (TZ1)  dcbl=Trip Zone 2 input (TZ2)  dcah_type2=GPTRIP1SEL/(TZ1)  dcal_type2=GPTRIP1SEL/(TZ1)  dcbh_type2=GPTRIP1SEL/(TZ1)  dcbl_type2=GPTRIP1SEL/(TZ1)  gendcaevt1=Event disabled  gendcaevt2=Event disabled  gendcbevt1=Event disabled  gendcbevt2=Event disabled  dcaevt1src=DCAEVT1 with sync  dcaevt2src=DCAEVT2 with sync  dcbevt1src=DCBEVT1 with sync  dcbevt2src=DCBEVT2 with sync  pulsesel=Counter equals to zero (CTR=Zero)  blankinv=off  blankoffset=0  blankwidth=0  evsrcsel=Filtered version of DCAEVT1 (DCAEVT1FILT)  encape=off
  wires:
  Timer Counter/1 -> Demux/1
  Demux/1 -> SW_A/1
  Demux/2 -> SW_B/1
  Demux/3 -> SW_C/1

== system genpath_firmware/ADC Interrupt Callback/Inverter Driver/Two Arm Modulation and First Quadrant Tracking Algorithm ==
  Phase Current : Inport
  Phase Voltage : Inport  Port=2
  DC Bus Voltage : Inport  Port=3
  Two Arm Modulation Enable : Inport  Port=4
  Upper Switch Duty Cycle : Inport  Port=5
  First Quadrant Tracking Algorithm : Subsystem
  Two Arm Modulation Algorithm : Subsystem
  Phase Voltage Out : Outport
  wires:
  Phase Voltage/1 -> Two Arm Modulation Algorithm/4(Phase Voltage), First Quadrant Tracking Algorithm/2(Phase Current)
  Phase Current/1 -> First Quadrant Tracking Algorithm/1(Phase Voltage)
  Two Arm Modulation Enable/1 -> Two Arm Modulation Algorithm/1(Enable)
  DC Bus Voltage/1 -> Two Arm Modulation Algorithm/2(DC Bus Voltage)
  First Quadrant Tracking Algorithm/1(Upper Switch Always Conduct) -> Two Arm Modulation Algorithm/3(Upper Switch Always Conduct)
  Two Arm Modulation Algorithm/1(Out1) -> Phase Voltage Out/1
  Upper Switch Duty Cycle/1 -> First Quadrant Tracking Algorithm/3(Enable)

== system genpath_firmware/ADC Interrupt Callback/MPPT Algorithm/Derivative ==
  In3 : Inport
  Gain : Gain  Gain=10e3
  Subtract : Sum  Inputs=+-
  Unit Delay : UnitDelay  SampleTime=-1  HasFrameUpgradeWarning=on
  Out1 : Outport
  wires:
  In3/1 -> Unit Delay/1, Subtract/1
  Unit Delay/1 -> Subtract/2
  Subtract/1 -> Gain/1
  Gain/1 -> Out1/1

== system genpath_firmware/ADC Interrupt Callback/Data Logger/Packet Serializer/Avoid Header and Terminator Collision ==
  Data Packet : Inport  Partition=on  PartitionDimension=1  PartitionWidth=1  PartitionOffset=0
  For Each : ForEach  DisableCoverage=on
  If Action Subsystem : Subsystem  TreatAsAtomicUnit=on
  If Action Subsystem1 : Subsystem  TreatAsAtomicUnit=on
  If Action Subsystem2 : Subsystem  TreatAsAtomicUnit=on
  If1 : If  IfExpression=u1 == 61166  ElseIfExpressions=u1 == 65535
  Merge : Merge  Inputs=3
  Data : Outport  ConcatenationDimension=1
  wires:
  Data Packet/1 -> If Action Subsystem2/1(Data Packet), If1/1
  If1/1 -> If Action Subsystem/Action
  If1/2 -> If Action Subsystem1/Action
  If Action Subsystem/1(Out1) -> Merge/1
  If Action Subsystem1/1(Out1) -> Merge/2
  If Action Subsystem2/1(Out1) -> Merge/3
  If1/3 -> If Action Subsystem2/Action
  Merge/1 -> Data/1

== system genpath_firmware/ADC Interrupt Callback/Data Logger/Packet Serializer/Data ==
  Data : Inport
  Data_width : Inport  Port=2
  Action Port : ActionPort  ActionPortLabel=else
  Mux : Mux  Inputs=3
  Start : Constant  Value=0  OutDataTypeStr=Inherit: Inherit via back propagation
  Start1 : Constant  Value=0  OutDataTypeStr=Inherit: Inherit via back propagation
  Data_out : Outport  VectorParamsAs1DForOutWhenUnconnected=off
  Iteration : Outport  Port=2  VectorParamsAs1DForOutWhenUnconnected=off
  wires:
  Start/1 -> Mux/2
  Mux/1 -> Data_out/1
  Data/1 -> Mux/1
  Data_width/1 -> Iteration/1
  Start1/1 -> Mux/3

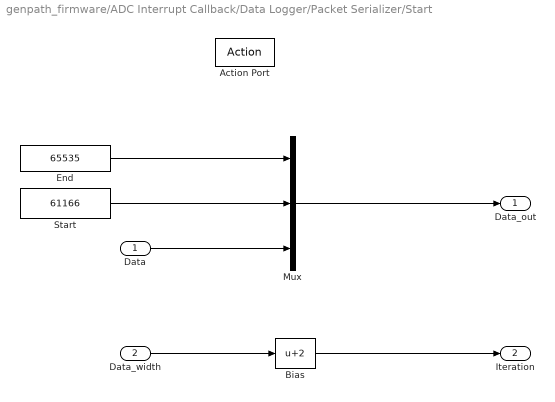
== system genpath_firmware/ADC Interrupt Callback/Data Logger/Packet Serializer/Start ==
  Data : Inport
  Data_width : Inport  Port=2
  Action Port : ActionPort  ActionPortLabel=if(u1 == 0)
  Bias : Bias  Bias=2
  End : Constant  Value=65535  OutDataTypeStr=Inherit: Inherit via back propagation
  Mux : Mux  Inputs=3
  Start : Constant  Value=61166  OutDataTypeStr=Inherit: Inherit via back propagation
  Data_out : Outport  VectorParamsAs1DForOutWhenUnconnected=off
  Iteration : Outport  Port=2  VectorParamsAs1DForOutWhenUnconnected=off
  wires:
  Mux/1 -> Data_out/1
  Data_width/1 -> Bias/1
  Bias/1 -> Iteration/1
  Data/1 -> Mux/3
  End/1 -> Mux/1
  Start/1 -> Mux/2

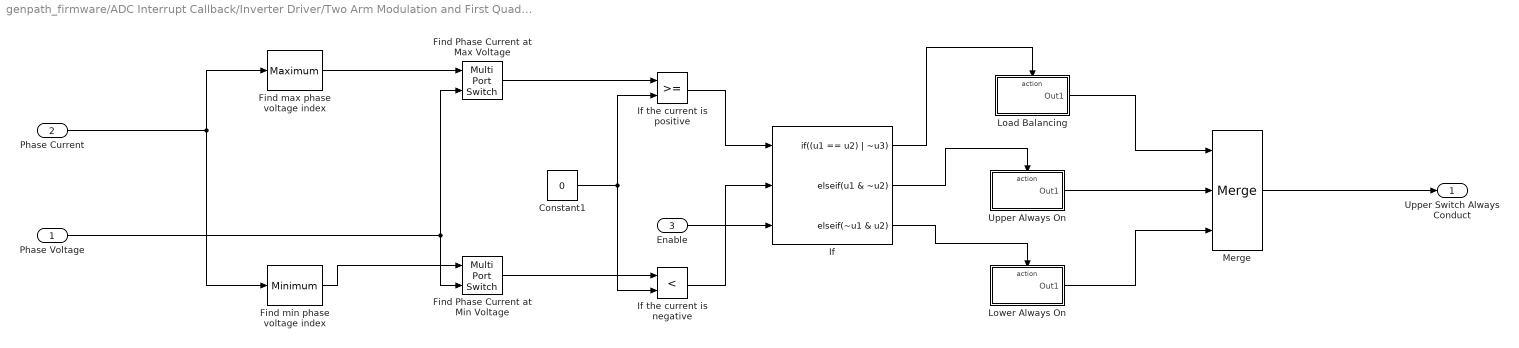
== system genpath_firmware/ADC Interrupt Callback/Inverter Driver/Two Arm Modulation and First Quadrant Tracking Algorithm/First Quadrant Tracking Algorithm ==
  Phase Voltage : Inport
  Phase Current : Inport  Port=2
  Enable : Inport  Port=3
  Constant1 : Constant  Value=0  OutDataTypeStr=Inherit: Inherit via back propagation
  "Find Phase Current at Max Voltage " : MultiPortSwitch  DataPortOrder=Zero-based contiguous  Inputs=1  zeroidx=on
  Find Phase Current at Min Voltage : MultiPortSwitch  DataPortOrder=Zero-based contiguous  Inputs=1  zeroidx=on
  Find max phase voltage index : dspstat3/Maximum  operation=maximum  fcn=Index  indexBase=Zero  operateOver=Each column  Dimension=1  InputProcessing=Columns as channels (frame based)  reset=None  roiEnable=off  roiType=Rectangles  roiPortion=Entire ROI  roiOutput=Individual statistics for each ROI  roiFlag=off  roundingMode=Floor  overflowMode=off  accumDataTypeStr=Inherit: Same as product output  accumLastDataTypeStr=Inherit: Same as product output
  Find min phase voltage index : dspstat3/Minimum  operation=minimum  fcn=Index  indexBase=Zero  operateOver=Each column  Dimension=1  InputProcessing=Columns as channels (frame based)  reset=None  roiEnable=off  roiType=Rectangles  roiPortion=Entire ROI  roiOutput=Individual statistics for each ROI  roiFlag=off  roundingMode=Floor  overflowMode=off
      settings: SourceProductBaseCode=DS
  If : If  NumInputs=3  IfExpression=(u1 == u2) | ~u3  ElseIfExpressions=u1 & ~u2,~u1 & u2  ShowElse=off
  If the current is negative : RelationalOperator  Operator=<  OutDataTypeStr=boolean  RndMeth=Simplest
  If the current is positive : RelationalOperator  OutDataTypeStr=boolean  RndMeth=Simplest
  Load Balancing : Subsystem  TreatAsAtomicUnit=on
  Lower Always On : Subsystem  TreatAsAtomicUnit=on
  Merge : Merge  Inputs=3
  Upper Always On : Subsystem  TreatAsAtomicUnit=on
  Upper Switch Always Conduct : Outport
  wires:
  If the current is negative/1 -> If/2
  Find max phase voltage index/1 -> "Find Phase Current at Max Voltage "/1
  Phase Voltage/1 -> "Find Phase Current at Max Voltage "/2, Find Phase Current at Min Voltage/2
  If/3 -> Lower Always On/Action
  Find min phase voltage index/1 -> Find Phase Current at Min Voltage/1
  Phase Current/1 -> Find max phase voltage index/1, Find min phase voltage index/1
  Constant1/1 -> If the current is negative/2, If the current is positive/2
  If/2 -> Upper Always On/Action
  "Find Phase Current at Max Voltage "/1 -> If the current is positive/1
  If/1 -> Load Balancing/Action
  Upper Always On/1(Out1) -> Merge/2
  Lower Always On/1(Out1) -> Merge/3
  If the current is positive/1 -> If/1
  Load Balancing/1(Out1) -> Merge/1
  Merge/1 -> Upper Switch Always Conduct/1
  Find Phase Current at Min Voltage/1 -> If the current is negative/1
  Enable/1 -> If/3

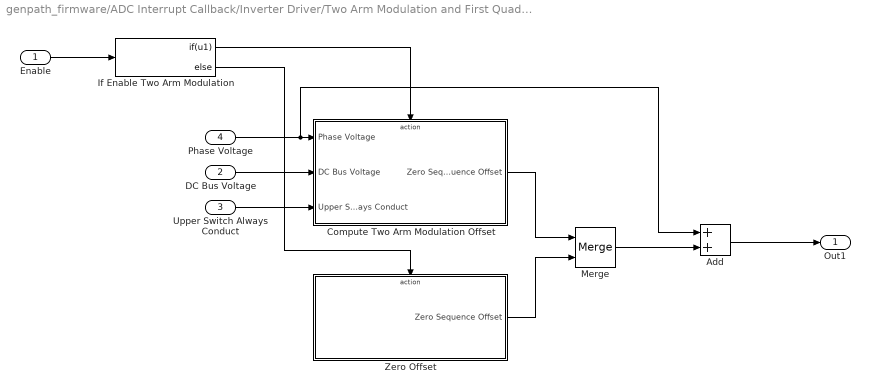
== system genpath_firmware/ADC Interrupt Callback/Inverter Driver/Two Arm Modulation and First Quadrant Tracking Algorithm/Two Arm Modulation Algorithm ==
  Enable : Inport
  DC Bus Voltage : Inport  Port=2
  Upper Switch Always Conduct : Inport  Port=3
  Phase Voltage : Inport  Port=4
  Add : Sum
  Compute Two Arm Modulation Offset : Subsystem
  If Enable Two Arm Modulation : If  IfExpression=u1
  Merge : Merge
  Zero Offset : Subsystem  TreatAsAtomicUnit=on
  Out1 : Outport
  wires:
  Phase Voltage/1 -> Add/1, Compute Two Arm Modulation Offset/1(Phase Voltage)
  Zero Offset/1(Zero Sequence Offset) -> Merge/2
  If Enable Two Arm Modulation/2 -> Zero Offset/Action
  Enable/1 -> If Enable Two Arm Modulation/1
  Compute Two Arm Modulation Offset/1(Zero Sequence Offset) -> Merge/1
  Merge/1 -> Add/2
  If Enable Two Arm Modulation/1 -> Compute Two Arm Modulation Offset/Action
  Add/1 -> Out1/1
  DC Bus Voltage/1 -> Compute Two Arm Modulation Offset/2(DC Bus Voltage)
  Upper Switch Always Conduct/1 -> Compute Two Arm Modulation Offset/3(Upper Switch Always Conduct)

== system genpath_firmware/ADC Interrupt Callback/Data Logger/Packet Serializer/Avoid Header and Terminator Collision/If Action Subsystem ==
  Action Port : ActionPort  ActionPortLabel=if(u1 == 61166)
  Constant : Constant  Value=258  OutDataTypeStr=Inherit: Inherit via back propagation
  Out1 : Outport
  wires:
  Constant/1 -> Out1/1

== system genpath_firmware/ADC Interrupt Callback/Data Logger/Packet Serializer/Avoid Header and Terminator Collision/If Action Subsystem1 ==
  Action Port : ActionPort  ActionPortLabel=elseif( u1 == 65535)
  Constant : Constant  Value=515  OutDataTypeStr=Inherit: Inherit via back propagation
  Out1 : Outport
  wires:
  Constant/1 -> Out1/1

== system genpath_firmware/ADC Interrupt Callback/Data Logger/Packet Serializer/Avoid Header and Terminator Collision/If Action Subsystem2 ==
  Data Packet : Inport
  Action Port : ActionPort  ActionPortLabel=else
  Out1 : Outport
  wires:
  Data Packet/1 -> Out1/1

== system genpath_firmware/ADC Interrupt Callback/Inverter Driver/Two Arm Modulation and First Quadrant Tracking Algorithm/First Quadrant Tracking Algorithm/Load Balancing ==
  Action Port : ActionPort  ActionPortLabel=if((u1 == u2) | ~u3)
  Constant : Constant  Value=250  OutDataTypeStr=Inherit: Inherit via back propagation
  Counter Limited : simulink/Sources/Counter Limited  uplimit=500  tsamp=-1
  Equal : RelationalOperator  OutDataTypeStr=boolean  RndMeth=Simplest  InputSameDT=on
  Out1 : Outport
  wires:
  Equal/1 -> Out1/1
  Constant/1 -> Equal/2
  Counter Limited/1 -> Equal/1

== system genpath_firmware/ADC Interrupt Callback/Inverter Driver/Two Arm Modulation and First Quadrant Tracking Algorithm/First Quadrant Tracking Algorithm/Lower Always On ==
  Action Port : ActionPort  ActionPortLabel=elseif(~u1 & u2)
  Constant : Constant  Value=false
  Out1 : Outport
  wires:
  Constant/1 -> Out1/1

== system genpath_firmware/ADC Interrupt Callback/Inverter Driver/Two Arm Modulation and First Quadrant Tracking Algorithm/First Quadrant Tracking Algorithm/Upper Always On ==
  Action Port : ActionPort  ActionPortLabel=elseif(u1 & ~u2)
  Constant : Constant  Value=true
  Out1 : Outport
  wires:
  Constant/1 -> Out1/1

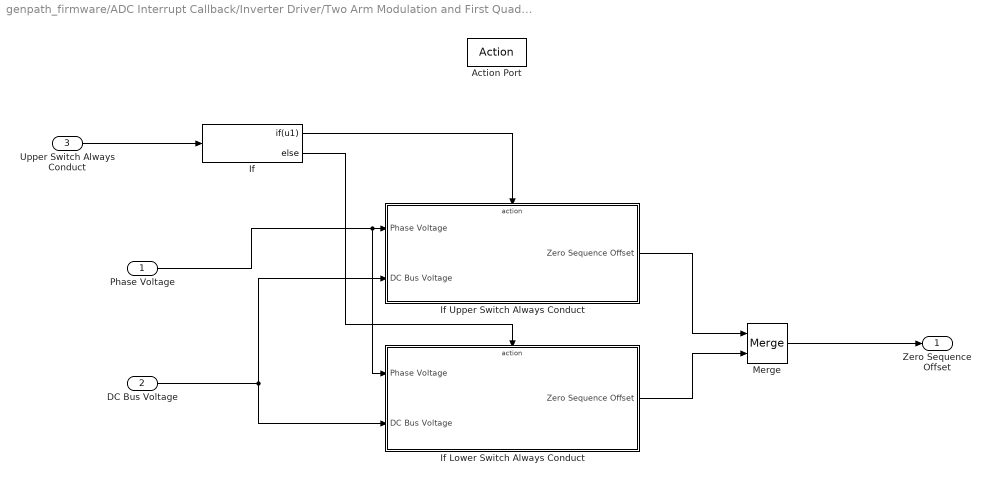
== system genpath_firmware/ADC Interrupt Callback/Inverter Driver/Two Arm Modulation and First Quadrant Tracking Algorithm/Two Arm Modulation Algorithm/Compute Two Arm Modulation Offset ==
  Phase Voltage : Inport
  DC Bus Voltage : Inport  Port=2
  Upper Switch Always Conduct : Inport  Port=3  OutDataTypeStr=boolean
  Action Port : ActionPort  ActionPortLabel=if(u1)
  If : If  IfExpression=u1
  If Lower Switch Always Conduct : Subsystem  TreatAsAtomicUnit=on
  If Upper Switch Always Conduct : Subsystem  TreatAsAtomicUnit=on
  Merge : Merge
  Zero Sequence Offset : Outport
  wires:
  Upper Switch Always Conduct/1 -> If/1
  If/1 -> If Upper Switch Always Conduct/Action
  If/2 -> If Lower Switch Always Conduct/Action
  Phase Voltage/1 -> If Lower Switch Always Conduct/1(Phase Voltage), If Upper Switch Always Conduct/1(Phase Voltage)
  DC Bus Voltage/1 -> If Lower Switch Always Conduct/2(DC Bus Voltage), If Upper Switch Always Conduct/2(DC Bus Voltage)
  If Upper Switch Always Conduct/1(Zero Sequence Offset) -> Merge/1
  If Lower Switch Always Conduct/1(Zero Sequence Offset) -> Merge/2
  Merge/1 -> Zero Sequence Offset/1

== system genpath_firmware/ADC Interrupt Callback/Inverter Driver/Two Arm Modulation and First Quadrant Tracking Algorithm/Two Arm Modulation Algorithm/Zero Offset ==
  Action Port : ActionPort  ActionPortLabel=else
  Ground : Ground
  Zero Sequence Offset : Outport
  wires:
  Ground/1 -> Zero Sequence Offset/1

== system genpath_firmware/ADC Interrupt Callback/Inverter Driver/Two Arm Modulation and First Quadrant Tracking Algorithm/Two Arm Modulation Algorithm/Compute Two Arm Modulation Offset/If Lower Switch Always Conduct ==
  Phase Voltage : Inport
  DC Bus Voltage : Inport  Port=2
  Action Port : ActionPort  ActionPortLabel=else
  Add : Sum  Inputs=--
  Gain : Gain  Gain=1/2
  Max : MinMax
  Zero Sequence Offset : Outport
  wires:
  Add/1 -> Zero Sequence Offset/1
  Phase Voltage/1 -> Max/1
  Max/1 -> Add/1
  DC Bus Voltage/1 -> Gain/1
  Gain/1 -> Add/2

== system genpath_firmware/ADC Interrupt Callback/Inverter Driver/Two Arm Modulation and First Quadrant Tracking Algorithm/Two Arm Modulation Algorithm/Compute Two Arm Modulation Offset/If Upper Switch Always Conduct ==
  Phase Voltage : Inport
  DC Bus Voltage : Inport  Port=2
  Action Port : ActionPort  ActionPortLabel=if(u1)
  Add : Sum  Inputs=-+
  Gain : Gain  Gain=1/2
  Max : MinMax  Function=max
  Zero Sequence Offset : Outport
  wires:
  Phase Voltage/1 -> Max/1
  Max/1 -> Add/1
  Add/1 -> Zero Sequence Offset/1
  DC Bus Voltage/1 -> Gain/1
  Gain/1 -> Add/2
